simulink model "FullAdder"  (R2016a)
settings: Solver=VariableStepAuto  StartTime=0.0  StopTime=10.0  RelTol=1e-3
settings Model: Creator=duyvu  LastModifiedBy=duyvu

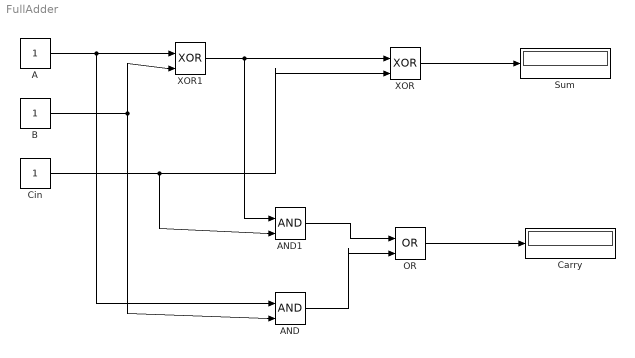
== system FullAdder ==
  A : Constant
  AND : Logic  IconShape=distinctive  AllPortsSameDT=off  OutDataTypeStr=boolean
  AND1 : Logic  IconShape=distinctive  AllPortsSameDT=off  OutDataTypeStr=boolean
  B : Constant
  Carry : Display
  Cin : Constant
  "OR " : Logic  Operator=OR  IconShape=distinctive  AllPortsSameDT=off  OutDataTypeStr=boolean
  Sum : Display
  XOR : Logic  Operator=XOR  IconShape=distinctive  AllPortsSameDT=off  OutDataTypeStr=boolean
  XOR1 : Logic  Operator=XOR  IconShape=distinctive  AllPortsSameDT=off  OutDataTypeStr=boolean
  wires:
  XOR/1 -> Sum/1
  XOR1/1 -> AND1/1, XOR/1
  A/1 -> XOR1/1, AND/1
  B/1 -> AND/2, XOR1/2
  Cin/1 -> XOR/2, AND1/2
  "OR "/1 -> Carry/1
  AND1/1 -> "OR "/1
  AND/1 -> "OR "/2
